simulink subsystem "IL"  (R2024a)
settings: Solver=VariableStepAuto  StartTime=0.0  StopTime=10.0  RelTol=1e-3
libraries: px4lib x15
settings Model: Creator=gurt1  LastModifiedBy=gurt1

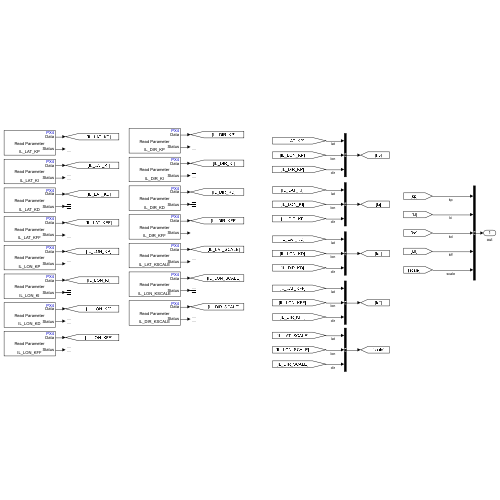
[thumbnail: Simulink's stored preview of the top-level diagram]
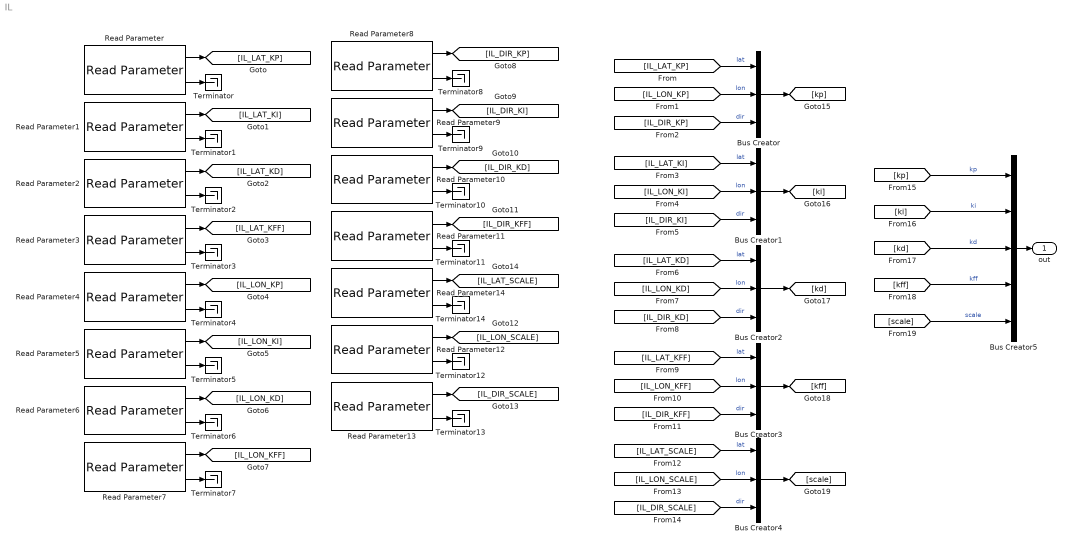
== system IL ==
  Bus Creator{,1..4} (5 alike) : BusCreator  Inputs=3
  Bus Creator5 : BusCreator  Inputs=5
  Read Parameter : px4lib/Read Parameter  ParameterName=IL_LAT_KP  DataType=FLOAT  SampleTime=-1
  Read Parameter1 : px4lib/Read Parameter  ParameterName=IL_LAT_KI  DataType=FLOAT  SampleTime=-1
  Read Parameter10 : px4lib/Read Parameter  ParameterName=IL_DIR_KD  DataType=FLOAT  SampleTime=-1
  Read Parameter11 : px4lib/Read Parameter  ParameterName=IL_DIR_KFF  DataType=FLOAT  SampleTime=-1
  Read Parameter12 : px4lib/Read Parameter  ParameterName=IL_LON_KSCALE  DataType=FLOAT  SampleTime=-1
  Read Parameter13 : px4lib/Read Parameter  ParameterName=IL_DIR_KSCALE  DataType=FLOAT  SampleTime=-1
  Read Parameter14 : px4lib/Read Parameter  ParameterName=IL_LAT_KSCALE  DataType=FLOAT  SampleTime=-1
  Read Parameter2 : px4lib/Read Parameter  ParameterName=IL_LAT_KD  DataType=FLOAT  SampleTime=-1
  Read Parameter3 : px4lib/Read Parameter  ParameterName=IL_LAT_KFF  DataType=FLOAT  SampleTime=-1
  Read Parameter4 : px4lib/Read Parameter  ParameterName=IL_LON_KP  DataType=FLOAT  SampleTime=-1
  Read Parameter5 : px4lib/Read Parameter  ParameterName=IL_LON_KI  DataType=FLOAT  SampleTime=-1
  Read Parameter6 : px4lib/Read Parameter  ParameterName=IL_LON_KD  DataType=FLOAT  SampleTime=-1
  Read Parameter7 : px4lib/Read Parameter  ParameterName=IL_LON_KFF  DataType=FLOAT  SampleTime=-1
  Read Parameter8 : px4lib/Read Parameter  ParameterName=IL_DIR_KP  DataType=FLOAT  SampleTime=-1
  Read Parameter9 : px4lib/Read Parameter  ParameterName=IL_DIR_KI  DataType=FLOAT  SampleTime=-1
  Terminator{,1..14} (15 alike) : Terminator
  out : Outport
  wires:
  [IL_LON_KFF] -> Bus Creator3/2  "lon"
  Read Parameter6/2 -> Terminator6/1
  Read Parameter12/2 -> Terminator12/1
  [IL_DIR_SCALE] -> Bus Creator4/3  "dir"
  [ki] -> Bus Creator5/2  "ki"
  Read Parameter13/1 -> [IL_DIR_SCALE]
  Read Parameter1/1 -> [IL_LAT_KI]
  Read Parameter1/2 -> Terminator1/1
  Read Parameter11/2 -> Terminator11/1
  Bus Creator1/1 -> [ki]
  Read Parameter/2 -> Terminator/1
  [scale] -> Bus Creator5/5  "scale"
  Read Parameter14/2 -> Terminator14/1
  [IL_LAT_KFF] -> Bus Creator3/1  "lat"
  Read Parameter/1 -> [IL_LAT_KP]
  Read Parameter3/2 -> Terminator3/1
  [IL_LON_KP] -> Bus Creator/2  "lon"
  Read Parameter6/1 -> [IL_LON_KD]
  Read Parameter13/2 -> Terminator13/1
  Read Parameter5/2 -> Terminator5/1
  [IL_LON_KD] -> Bus Creator2/2  "lon"
  Read Parameter4/2 -> Terminator4/1
  [IL_DIR_KP] -> Bus Creator/3  "dir"
  Read Parameter7/1 -> [IL_LON_KFF]
  Read Parameter2/1 -> [IL_LAT_KD]
  [IL_LAT_KI] -> Bus Creator1/1  "lat"
  [IL_DIR_KFF] -> Bus Creator3/3  "dir"
  Read Parameter2/2 -> Terminator2/1
  [IL_LAT_KP] -> Bus Creator/1  "lat"
  Read Parameter7/2 -> Terminator7/1
  Read Parameter4/1 -> [IL_LON_KP]
  Read Parameter5/1 -> [IL_LON_KI]
  Bus Creator5/1 -> out/1
  Read Parameter11/1 -> [IL_DIR_KFF]
  Read Parameter3/1 -> [IL_LAT_KFF]
  Read Parameter9/2 -> Terminator9/1
  Read Parameter10/1 -> [IL_DIR_KD]
  Read Parameter9/1 -> [IL_DIR_KI]
  Bus Creator2/1 -> [kd]
  Read Parameter8/1 -> [IL_DIR_KP]
  Read Parameter12/1 -> [IL_LON_SCALE]
  [IL_DIR_KD] -> Bus Creator2/3  "dir"
  Read Parameter8/2 -> Terminator8/1
  [IL_LAT_KD] -> Bus Creator2/1  "lat"
  [IL_LON_SCALE] -> Bus Creator4/2  "lon"
  Read Parameter10/2 -> Terminator10/1
  [kd] -> Bus Creator5/3  "kd"
  Read Parameter14/1 -> [IL_LAT_SCALE]
  Bus Creator3/1 -> [kff]
  [IL_DIR_KI] -> Bus Creator1/3  "dir"
  Bus Creator/1 -> [kp]
  [IL_LON_KI] -> Bus Creator1/2  "lon"
  [kff] -> Bus Creator5/4  "kff"
  [IL_LAT_SCALE] -> Bus Creator4/1  "lat"
  Bus Creator4/1 -> [scale]
  [kp] -> Bus Creator5/1  "kp"
